simulink model "Task5_OutputFeedback_LTR"  (R2024b)
settings: Solver=ode45  StartTime=0.0  StopTime=80  MaxStep=0.005  RelTol=1e-7  AbsTol=1e-9
settings Model: Creator=LAPTOPASADI  LastModifiedBy=LAPTOPASADI
settings DataIOCC: SaveOutput=off  SignalLogging=off  DSMLogging=off  SaveTime=off  ReturnWorkspaceOutputs=off

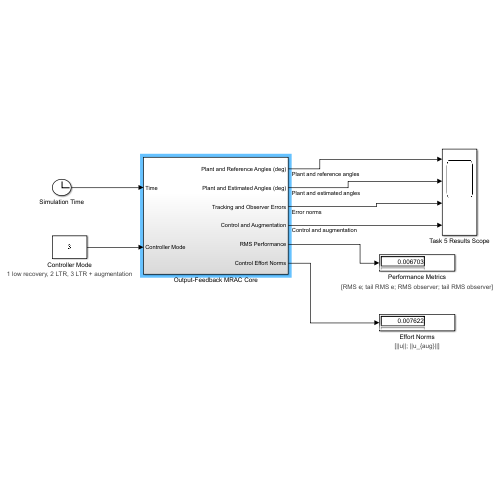
[thumbnail: Simulink's stored preview of the top-level diagram]
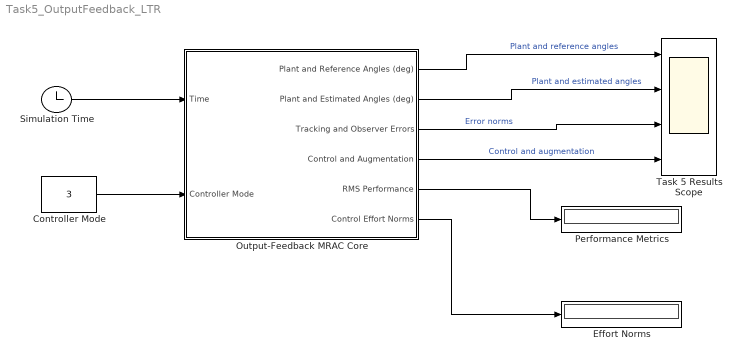
== system Task5_OutputFeedback_LTR ==
  Controller Mode : Constant  Value=3  OutDataTypeStr=double
      settings: AttributesFormatString=1 low recovery, 2 LTR, 3 LTR + augmentation
  Effort Norms : Display
      settings: AttributesFormatString=[||u||; ||u_{aug}||]
  Output-Feedback MRAC Core : Subsystem
  Performance Metrics : Display
      settings: AttributesFormatString=[RMS e; tail RMS e; RMS observer; tail RMS observer]
  Simulation Time : Clock
  Task 5 Results Scope : Scope  NumInputPorts=4
  wires:
  Simulation Time/1 -> Output-Feedback MRAC Core/1(Time)
  Controller Mode/1 -> Output-Feedback MRAC Core/2(Controller Mode)
  Output-Feedback MRAC Core/1(Plant and Reference Angles (deg)) -> Task 5 Results Scope/1  "Plant and reference angles"
  Output-Feedback MRAC Core/2(Plant and Estimated Angles (deg)) -> Task 5 Results Scope/2  "Plant and estimated angles"
  Output-Feedback MRAC Core/3(Tracking and Observer Errors) -> Task 5 Results Scope/3  "Error norms"
  Output-Feedback MRAC Core/4(Control and Augmentation) -> Task 5 Results Scope/4  "Control and augmentation"
  Output-Feedback MRAC Core/5(RMS Performance) -> Performance Metrics/1
  Output-Feedback MRAC Core/6(Control Effort Norms) -> Effort Norms/1

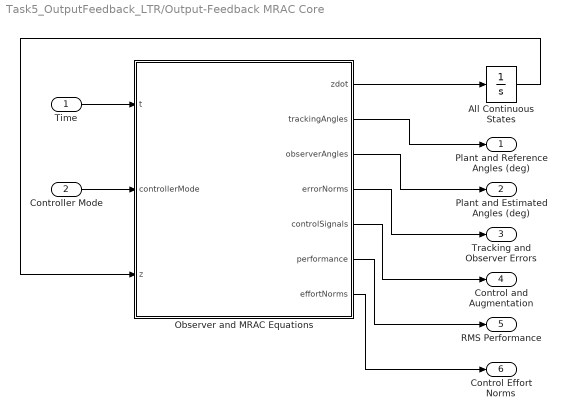
== system Task5_OutputFeedback_LTR/Output-Feedback MRAC Core ==
  Time : Inport
  Controller Mode : Inport  Port=2
  All Continuous States : Integrator  InitialCondition=[0;0;0;0;0;0;0;0;0;0;0;0;0;0;0;0;0;0;0;-0.66823529411764704;0;0;-0.66823529411764704;0;-0.093784508916032808;0;-0.084095775670305087;-0.093784508916032808;0;-0.084095775670305087;-0.020546127010358625;0;0.38386217602841338;-0.020546127010358625;0;0.38386217602841338;0;0.66823529411764704;0;0.093784508916032808;0;0.084095775670305087;0.020546127010358625;0;-0.38386217602841338;0;0.15647058823529411;0;0;-0.0016705882352941175;0;-0.018538798274099509;0;-0.011825968453636653;-0.00023446127229008202;0;-0.00021023943917576274;-0.0040614437113499612;0;0.053980618503995631;-5.1365317525896568e-05;0;0.00095965544007103345;0;0;0;0;0;0;0;0;0;0;0;0;0;0;0;0]
  Observer and MRAC Equations : MATLAB Function  TreatAsAtomicUnit=on
  Plant and Reference Angles (deg) : Outport
  Plant and Estimated Angles (deg) : Outport  Port=2
  Tracking and Observer Errors : Outport  Port=3
  Control and Augmentation : Outport  Port=4
  RMS Performance : Outport  Port=5
  Control Effort Norms : Outport  Port=6
  wires:
  Time/1 -> Observer and MRAC Equations/1(t)
  Controller Mode/1 -> Observer and MRAC Equations/2(controllerMode)
  Observer and MRAC Equations/4(errorNorms) -> Tracking and Observer Errors/1
  Observer and MRAC Equations/1(zdot) -> All Continuous States/1
  Observer and MRAC Equations/2(trackingAngles) -> Plant and Reference Angles (deg)/1
  Observer and MRAC Equations/3(observerAngles) -> Plant and Estimated Angles (deg)/1
  Observer and MRAC Equations/5(controlSignals) -> Control and Augmentation/1
  Observer and MRAC Equations/6(performance) -> RMS Performance/1
  Observer and MRAC Equations/7(effortNorms) -> Control Effort Norms/1
  All Continuous States/1 -> Observer and MRAC Equations/3(z)

== matlab function Task5_OutputFeedback_LTR/Output-Feedback MRAC Core/Observer and MRAC Equations ==
  data: t input; zdot output; controllerMode input; z input; trackingAngles output; observerAngles output; errorNorms output; controlSignals output; performance output; effortNorms output
function [zdot,trackingAngles,observerAngles,errorNorms,controlSignals,performance,effortNorms] = outputFeedbackMRAC(t,controllerMode,z)
%#codegen
% Standalone Task 5 equations. The three modes share the same plant and command.

x = z(1:6);
xm = z(7:12);
xhat = z(13:18);
KxHat = reshape(z(19:36),6,3);
KrHat = reshape(z(37:45),3,3);
ThetaHat = reshape(z(46:63),6,3);
WHat = reshape(z(64:75),4,3);
integrals = z(76:79);

G = [0,40.697674418604649,8.9159670109220599; ...
     5.9859154929577469,0,0; ...
     0,2.1783328492593665,-9.9431818181818166];
A = [zeros(3),eye(3);zeros(3),zeros(3)];
B = [zeros(3);G];
Am = [zeros(3),eye(3);-4*eye(3),-4*eye(3)];
Bm = [zeros(3);4*eye(3)];
C = [eye(3),zeros(3)];
P = [1.125,0,0,0.125,0,0; ...
     0,1.125,0,0,0.125,0; ...
     0,0,1.125,0,0,0.125; ...
     0.125,0,0,0.15625,0,0; ...
     0,0.125,0,0,0.15625,0; ...
     0,0,0.125,0,0,0.15625];
ThetaPlantT = [0,0.15647058823529411,0,0,-0.0016705882352941175,0; ...
    -0.018538798274099509,0,-0.011825968453636653,-0.00023446127229008202,0,-0.00021023943917576274; ...
    -0.0040614437113499612,0,0.053980618503995631,-0.000051365317525896568,0,0.00095965544007103345];
WtrueT = [0.0030,-0.0010,0.0015,0.0020; ...
         -0.0010,0.0025,-0.0010,0.0015; ...
          0.0010,-0.0015,0.0030,-0.0020];

Lbaseline = [2.8866202178607456,0,0; ...
             0,1.0941598462649884,0; ...
             0,0,1.4268151830472224; ...
             4.1662876410812055,0,0; ...
             0,0.59859238458931197,0; ...
             0,0,1.0179002832870401];
Lltr = [28.866200048092093,0,0; ...
        0,10.941586305278673,0; ...
        0,0,14.268144918865904; ...
        416.62875210823307,0,0; ...
        0,59.859154937930732,0; ...
        0,0,101.7899792128794];

if controllerMode < 1.5
    L = Lbaseline;
    augmentationEnabled = false;
else
    L = Lltr;
    augmentationEnabled = controllerMode >= 2.5;
end

reference = zeros(3,1);
if t >= 1
    tau = t-1;
    weights = [0.30,0.24,0.19,0.15,0.12];
    peaks = (pi/180)*[10;10;15];
    amplitude = peaks*weights;
    frequency = [0.31,0.53,0.79,1.07,1.37; ...
                 0.37,0.61,0.89,1.19,1.43; ...
                 0.43,0.67,0.97,1.27,1.51];
    reference = sum(amplitude.*sin(frequency*tau),2);
end

noiseAmplitude = (pi/180)*[0.002;0.002;0.003];
noiseFrequency = [7.3;8.1;9.2];
noisePhase = [0;0.7;1.3];
measurementNoise = noiseAmplitude.*sin(noiseFrequency*t+noisePhase);
measurement = C*x+measurementNoise;
innovation = measurement-C*xhat;

pHat = xhat(4); qHat = xhat(5); rHat = xhat(6);
phiHat = [qHat*rHat;pHat*rHat;pHat*qHat;pHat;qHat;rHat];
controllerError = xhat-xm;
adaptationSignal = controllerError.'*P*B;
psiHat = [sin(2*xhat(1));sin(2*xhat(2));sin(2*xhat(3));1];

uAug = zeros(3,1);
WHatDot = zeros(4,3);
if augmentationEnabled
    uAug = -WHat.'*psiHat;
    leakage = 0.005*norm(controllerError);
    WHatDot = 5*psiHat*adaptationSignal-5*leakage*WHat;
end
u = KxHat.'*xhat+KrHat.'*reference-ThetaHat.'*phiHat+uAug;

p = x(4); q = x(5); rBody = x(6);
phiTrue = [q*rBody;p*rBody;p*q;p;q;rBody];
psiTrue = [sin(2*x(1));sin(2*x(2));sin(2*x(3));1];
xdot = A*x+B*(u+ThetaPlantT*phiTrue+WtrueT*psiTrue);
xmdot = Am*xm+Bm*reference;
xhatDot = A*xhat+B*u+L*innovation;
KxHatDot = -50*xhat*adaptationSignal;
KrHatDot = -50*reference*adaptationSignal;
ThetaHatDot = 50*phiHat*adaptationSignal;

trackingError = x-xm;
observerError = x-xhat;
integralDot = [trackingError.'*trackingError;observerError.'*observerError;0;0];
if t >= 65
    integralDot(3) = trackingError.'*trackingError;
    integralDot(4) = observerError.'*observerError;
end
zdot = [xdot;xmdot;xhatDot;KxHatDot(:);KrHatDot(:); ...
        ThetaHatDot(:);WHatDot(:);integralDot];

trackingAngles = (180/pi)*[x(1:3);xm(1:3)];
observerAngles = (180/pi)*[x(1:3);xhat(1:3)];
errorNorms = [norm(trackingError);norm(observerError);norm(controllerError)];
controlSignals = [u;uAug];
elapsed = max(t,1e-9);
tailElapsed = max(t-65,1e-9);
performance = [sqrt(max(integrals(1),0)/elapsed); ...
               sqrt(max(integrals(3),0)/tailElapsed); ...
               sqrt(max(integrals(2),0)/elapsed); ...
               sqrt(max(integrals(4),0)/tailElapsed)];
effortNorms = [norm(u);norm(uAug)];
end
